simulink model "KF_e"  (R2018a)
settings: Solver=ode45  StartTime=0.0  StopTime=500  RelTol=1e-3  EnableMultiTasking=on
values from neighbouring files (symbols this model uses):
  K_pd = w_c*abs(1+w_c*T_f*i)/K    [KalmanFilter_d.m]    (also in KalmanFilter_e.m = w_c*abs(1+w_c*T_f*i)/K-0.2; KalmanFilter_f.m = w_c*abs(1+w_c*T_f*i)/K-0.2)
  T_d = T    (= 72.4391)    [KalmanFilter_d.m]    (also in KalmanFilter_e.m; KalmanFilter_f.m)
  T_f = tan(40/180*pi)/w_c    [KalmanFilter_d.m]    (also in KalmanFilter_e.m; KalmanFilter_f.m)
libraries: simulink x2
settings Model: Creator=markh  LastModifiedBy=hongyuz
settings DataIOCC: LimitDataPoints=on  SaveFormat=Array  SignalLoggingSaveFormat=ModelDataLogs  SignalLoggingName=sigsOut
settings OptimizationCC: InitFltsAndDblsToZero=on  LifeSpan=inf
settings DebuggingCC: SaveWithParameterizedLinksMsg=none  UnderspecifiedInitializationDetection=Classic  MergeDetectMultiDrivingBlocksExec=none  SignalResolutionControl=TryResolveAllWithWarning  MultiTaskDSMMsg=warning  MultiTaskCondExecSysMsg=none  FcnCallInpInsideContextMsg=warning  StateNameClashWarn=warning  SFUnexpectedBacktrackingDiag=warning  SFNoUnconditionalDefaultTransitionDiag=warning  SFExecutionAtInitializationDiag=none
settings HardwareCC: ProdBitPerPointer=32  ProdBitPerSizeT=32  ProdBitPerPtrDiffT=32  ProdLargestAtomicFloat=None  ProdIntDivRoundTo=Undefined  ProdEndianess=Unspecified  ProdWordSize=32  ProdHWDeviceType=32-bit Generic  TargetUnknown=on
settings ModelReferenceCC: PropagateSignalLabelsOutOfModel=off
settings RTWCC: Description=Generic Real-Time Target
settings CodeAppCC: StateflowObjectComments=on
settings GRTTargetCC: TargetFcnLib=ansi_tfl_tmw.mat  TargetLangStandard=C89/C90 (ANSI)  GeneratePreprocessorConditionals=Disable all  CombineOutputUpdateFcns=off  GRTInterface=on
settings ConfigComp: CovMetricSettings=dw  CovHtmlReporting=on  CovSaveCumulativeToWorkspaceVar=on  CovSaveSingleToWorkspaceVar=on  CovExternalEMLEnable=off

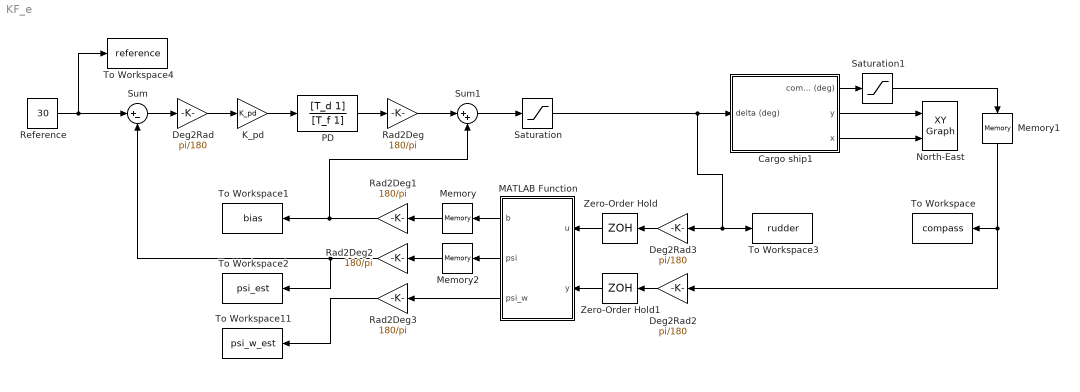
== system KF_e ==
  Cargo ship1 : Subsystem  mask(Simple shipmodel for a cargo ship){noise=on, current=on, logic=on}
      mask prompts: noise "measurement noise"; logic "waves"
      mask help:
      | Measurement noise:
      | 	checked = noise on
      | 	unchecked = noise off
      |
      | Current:
      | 	checked = current on
      | 	unchecked = current off
      |
      | Waves:
      | 	checked = waves on
      | 	unchecked = waves off
      |
      | Author: Jørgen Spjøtvold, 9/10-2003
      | TTK 4115 Linear system theory.
      | Modified by Jostein Bakkeheim 26/10-2006
  Deg2Rad : Gain  Gain=pi/180
  Deg2Rad2 : Gain  Gain=pi/180
  Deg2Rad3 : Gain  Gain=pi/180
  K_pd : Gain  Gain=K_pd
  MATLAB Function : MATLAB Function  TreatAsAtomicUnit=on
  Memory : Memory
  Memory1 : Memory
  Memory2 : Memory
  North-East : simulink/Sinks/XY Graph  xmin=-5000  xmax=5000  ymin=-5000  ymax=5000  st=-1
  PD : TransferFcn  Numerator=[T_d 1]  Denominator=[T_f 1]
  Rad2Deg{,1..3} (4 alike) : Gain  Gain=180/pi
  Reference : Constant  Value=30
  Saturation : Saturate  UpperLimit=45  LowerLimit=-45
  Saturation1 : Saturate  UpperLimit=35  LowerLimit=-35
  Sum : Sum  Inputs=|+-
  Sum1 : Sum  Inputs=|++
  To Workspace : ToWorkspace  VariableName=compass  SaveFormat=Timeseries  SampleTime=-1
  To Workspace1 : ToWorkspace  VariableName=bias  SaveFormat=Timeseries  SampleTime=-1
  To Workspace11 : ToWorkspace  VariableName=psi_w_est  SaveFormat=Timeseries  SampleTime=-1
  To Workspace2 : ToWorkspace  VariableName=psi_est  SaveFormat=Timeseries  SampleTime=-1
  To Workspace3 : ToWorkspace  VariableName=rudder  SaveFormat=Timeseries  SampleTime=-1
  To Workspace4 : ToWorkspace  VariableName=reference  SaveFormat=Timeseries  SampleTime=-1
  Zero-Order Hold : ZeroOrderHold  SampleTime=0.1
  Zero-Order Hold1 : ZeroOrderHold  SampleTime=0.1
  wires:
  K_pd/1 -> PD/1
  Deg2Rad/1 -> K_pd/1
  PD/1 -> Rad2Deg/1
  Sum/1 -> Deg2Rad/1
  Rad2Deg/1 -> Sum1/1
  Sum1/1 -> Saturation/1
  Reference/1 -> Sum/1, To Workspace4/1
  Memory/1 -> Rad2Deg1/1
  Saturation1/1 -> Memory1/1
  Rad2Deg1/1 -> Sum1/2, To Workspace1/1
  Rad2Deg2/1 -> To Workspace2/1, Sum/2
  Saturation/1 -> To Workspace3/1, Deg2Rad3/1, Cargo ship1/1(delta (deg))
  Memory1/1 -> Deg2Rad2/1, To Workspace/1
  Deg2Rad2/1 -> Zero-Order Hold1/1
  Deg2Rad3/1 -> Zero-Order Hold/1
  Cargo ship1/1(compass (deg)) -> Saturation1/1
  Cargo ship1/2(y) -> North-East/1
  Cargo ship1/3(x) -> North-East/2
  Zero-Order Hold/1 -> MATLAB Function/1(u)
  Zero-Order Hold1/1 -> MATLAB Function/2(y)
  MATLAB Function/1(b) -> Memory/1
  Memory2/1 -> Rad2Deg2/1
  Rad2Deg3/1 -> To Workspace11/1
  MATLAB Function/2(psi) -> Memory2/1
  MATLAB Function/3(psi_w) -> Rad2Deg3/1

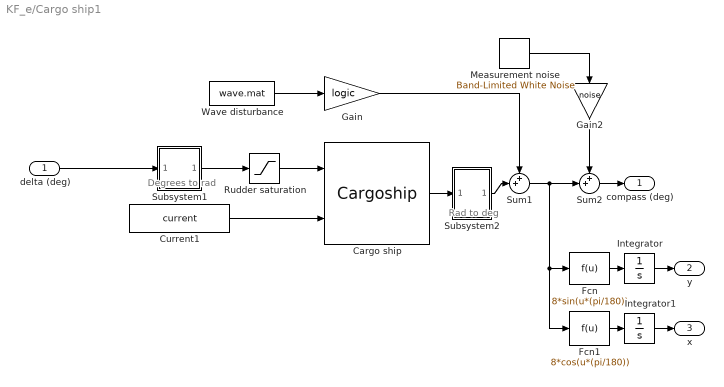
== system KF_e/Cargo ship1 ==
  note: Degrees to rad
  note: Rad to deg
  delta (deg) : Inport
  Cargo ship : S-Function  FunctionName=Cargoship  SFunctionDeploymentMode=off  EnableBusSupport=off  mask(Cargo ship){}
      mask help:
      | S-function which simulates a cargo ship.
      |
      | Author: Jørgen Spjøtvold
      | 20.10-2003
      | Modified by Jostein Bakkeheim 27.10.2006
  Current1 : Constant  Value=current
  Fcn : Fcn  Expr=8*sin(u*(pi/180))
  Fcn1 : Fcn  Expr=8*cos(u*(pi/180))
  Gain : Gain  Gain=logic  SaturateOnIntegerOverflow=on  OutDataTypeStr=Inherit: Same as input  ParamDataTypeStr=Inherit: Same as input
  Gain2 : Gain  Gain=noise  SaturateOnIntegerOverflow=on  OutDataTypeStr=Inherit: Same as input  ParamDataTypeStr=Inherit: Same as input
  Integrator : Integrator
  Integrator1 : Integrator
  Measurement noise : simulink/Sources/Band-Limited White Noise  Cov=[0.001]  Ts=.5  seed=[23341]
  Rudder saturation : Saturate  UpperLimit=45*(pi/180)  LowerLimit=-45*(pi/180)
  Subsystem1 : Subsystem  mask(degrees to radians){}
      mask help: Converts degrees to radians
      mask Display: fprintf('D2R');
  Subsystem2 : Subsystem  mask(radians to degrees){}
      mask help: Converts radians to degrees
      mask Display: fprintf('R2D');
  Sum1 : Sum  Inputs=++|  SaturateOnIntegerOverflow=on
  Sum2 : Sum  Inputs=++|  SaturateOnIntegerOverflow=on
  Wave disturbance : FromFile  FileName=wave.mat  SampleTime=0
  compass (deg) : Outport
  y : Outport  Port=2
  x : Outport  Port=3
  wires:
  delta (deg)/1 -> Subsystem1/1(In1)
  Fcn/1 -> Integrator/1
  Integrator/1 -> y/1
  Fcn1/1 -> Integrator1/1
  Integrator1/1 -> x/1
  Wave disturbance/1 -> Gain/1
  Subsystem2/1(Out1) -> Sum1/2
  Gain/1 -> Sum1/1
  Sum1/1 -> Fcn/1, Fcn1/1, Sum2/2
  Cargo ship/1 -> Subsystem2/1(In1)
  Subsystem1/1(Out1) -> Rudder saturation/1
  Rudder saturation/1 -> Cargo ship/1
  Sum2/1 -> compass (deg)/1
  Measurement noise/1 -> Gain2/1
  Gain2/1 -> Sum2/1
  Current1/1 -> Cargo ship/2

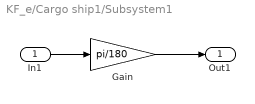
== system KF_e/Cargo ship1/Subsystem1 ==
  In1 : Inport
  Gain : Gain  Gain=pi/180  SaturateOnIntegerOverflow=on  OutDataTypeStr=Inherit: Same as input  ParamDataTypeStr=Inherit: Same as input
  Out1 : Outport
  wires:
  Gain/1 -> Out1/1
  In1/1 -> Gain/1

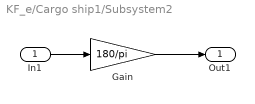
== system KF_e/Cargo ship1/Subsystem2 ==
  In1 : Inport
  Gain : Gain  Gain=180/pi  SaturateOnIntegerOverflow=on  OutDataTypeStr=Inherit: Same as input  ParamDataTypeStr=Inherit: Same as input
  Out1 : Outport
  wires:
  Gain/1 -> Out1/1
  In1/1 -> Gain/1

== matlab function KF_e/MATLAB Function ==
  data: b output; u input; psi output; y input; data parameter; psi_w output
function [b,psi,psi_w] = KF(u, y, data)
%#codegen
persistent init_flag A B C E Q R P_ x_ I

if (isempty(init_flag))
    
init_flag = 1;

% Initialization for system
[A,B,C,E,Q,R,P_,x_,I] = deal(data.Ad,data.Bd,data.Cd,data.Ed, ...
    data.Q, data.R, data.P_0, data.x_0, data.I);
% A=data.Ad;
% B=data.Bd;
% C=data.Cd;
% E=data.Ed;
% R=data.R;
% Q=data.Q;
% x_=data.x_0;
% P_=data.P_0;
% I=data.I;

end

% Compute the Kalman Gain
K = (P_*C')*inv((C*P_*C'+R));
% Update estimate with measurment
x_est = x_+K*(y-C*x_);
% Update error covariance matrix
P_est = (I-K*C)*P_*(I-K*C)'+K*R*K';
% Projet ahead
x_ = A*x_est+B*u;
P_ = A*P_est*A'+E*Q*E';

psi_w = x_est(2);
psi = x_est(3);
b = x_est(5);

end
